simulink library "motorLib"  (R2020b)
settings: Solver=VariableStepAuto  StartTime=0.0  StopTime=10.0  RelTol=1e-3
undefined symbols (not defined in the file): Controller
libraries: sharedutil x1
settings Model: Creator=dbell44  LastModifiedBy=dbell44

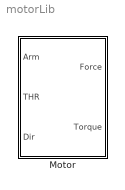
== system motorLib ==
  Motor : Subsystem

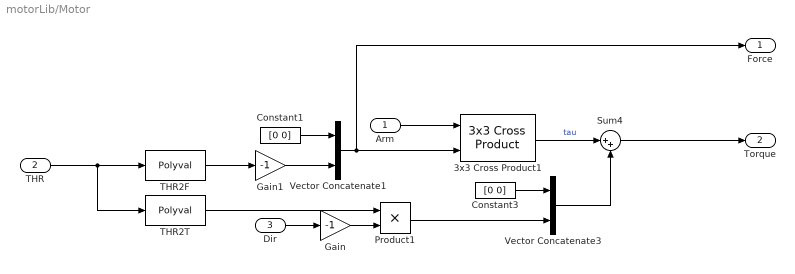
== system motorLib/Motor ==
  Arm : Inport
  THR : Inport  Port=2
  Dir : Inport  Port=3
  3x3 Cross Product1 : sharedutil/3x3 Cross Product  aMode=aMode
      settings: SourceProductBaseCode=AE,PW,MT,VE,VP
  Constant1 : Constant  Value=[0 0]
  Constant3 : Constant  Value=[0 0]
  Gain : Gain  Gain=-1
  Gain1 : Gain  Gain=-1
  Product1 : Product
  Sum4 : Sum  Inputs=|++
  THR2F : Polyval  Coefs=Controller.Throttle2F
  THR2T : Polyval  Coefs=Controller.Throttle2T
  Vector Concatenate1 : Concatenate  Mode=Multidimensional array
  Vector Concatenate3 : Concatenate  Mode=Multidimensional array
  Force : Outport
  Torque : Outport  Port=2
  wires:
  Constant3/1 -> Vector Concatenate3/1
  THR2T/1 -> Product1/1
  Sum4/1 -> Torque/1
  3x3 Cross Product1/1 -> Sum4/1  "tau"
  THR2F/1 -> Gain1/1
  Arm/1 -> 3x3 Cross Product1/1
  Constant1/1 -> Vector Concatenate1/1
  Gain1/1 -> Vector Concatenate1/2
  Vector Concatenate1/1 -> Force/1, 3x3 Cross Product1/2
  Dir/1 -> Gain/1
  Gain/1 -> Product1/2
  Product1/1 -> Vector Concatenate3/2
  Vector Concatenate3/1 -> Sum4/2
  THR/1 -> THR2F/1, THR2T/1
